simulink model "test_2d"  (R2014b)
settings: Solver=FixedStepDiscrete  StartTime=0.0  StopTime=10.0  FixedStep=1e-3  RelTol=1e-3
libraries: simulink x2, NDTable x1
settings Model: Creator=Torsten.Sommer  LastModifiedBy=Torsten.Sommer

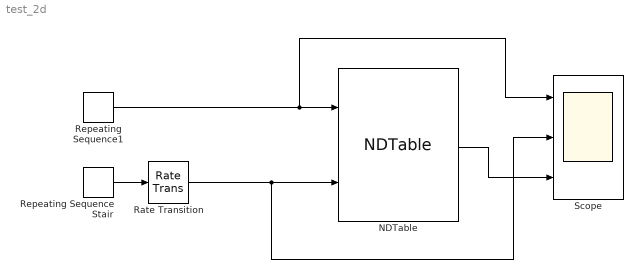
== system test_2d ==
  NDTable : NDTable/NDTable  filename='diode.sdf'  dataset='/I_f'  interp_method=Linear  extrap_method=Linear
  Rate Transition : RateTransition
  Repeating Sequence Stair : simulink/Sources/Repeating Sequence Stair  OutValues=[289.15 398.15 423.15]  tsamp=1  OutMin=[]  OutMax=[]  OutDataTypeStr=double  OutputDataTypeScalingMode=double  OutDataType=fixdt(0,8)  ConRadixGroup=Best Precision: Vector-wise  OutScaling=2^-12
  Repeating Sequence1 : simulink/Sources/Repeating Sequence  rep_seq_t=[0 1]  rep_seq_y=[0 1.92]
  Scope : Scope  NumInputPorts=3
      settings: TimeRange=10  YMin=0~0~-500  YMax=2~450~2000
  wires:
  NDTable/1 -> Scope/3
  Repeating Sequence Stair/1 -> Rate Transition/1
  Repeating Sequence1/1 -> Scope/1, NDTable/1
  Rate Transition/1 -> Scope/2, NDTable/2
